simulink model "inv_pend_delay"  (Simulink 8.6)
settings: Solver=ode45  StartTime=0.0  StopTime=2  RelTol=1e-3
settings Model: Creator=mengg_000  LastModifiedBy=Martin
settings DebuggingCC: FcnCallInpInsideContextMsg=UseLocalSettings

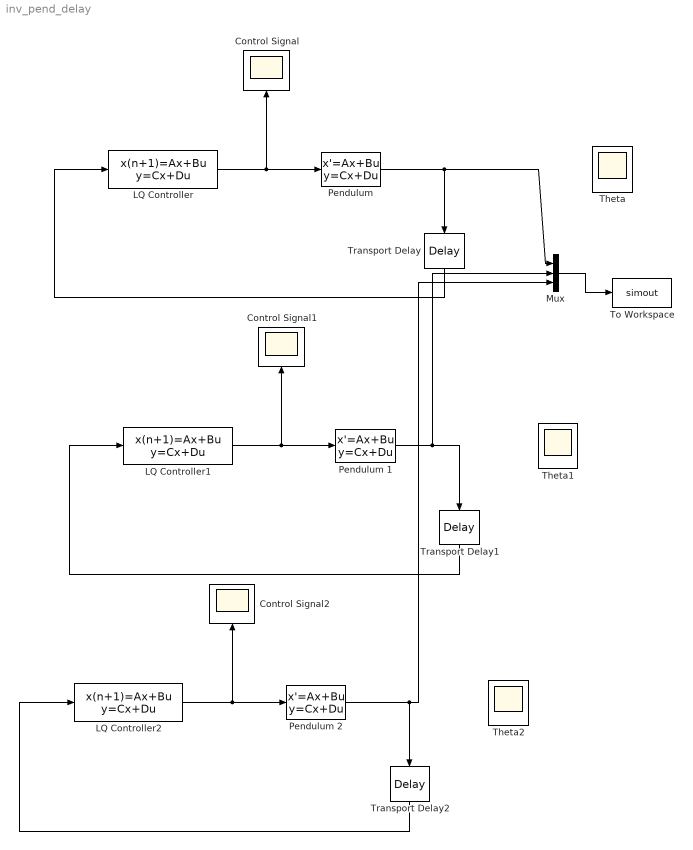
== system inv_pend_delay ==
  Control Signal : Scope
  Control Signal1 : Scope
  Control Signal2 : Scope
  LQ Controller : DiscreteStateSpace  A=|  B=|  C="[-12.1798  -13.3262         0]"  D=-8.1263  X0="[0;    0;   0]"  SampleTime=0.02
      A=|
      | [0.0389   -1.5001         0;
      |     0.0828    0.3594         0;
      |   -12.1798  -13.3262         0]
      B=|
      | [ -0.4344;
      |     0.1355;
      |    -8.1263]
  LQ Controller1 : DiscreteStateSpace  A=|  B=|  C="[-12.1798  -13.3262         0]"  D=-8.1263  X0="[0;    0;   0]"  SampleTime=0.02
      A=|
      | [0.0389   -1.5001         0;
      |     0.0828    0.3594         0;
      |   -12.1798  -13.3262         0]
      B=|
      | [ -0.4344;
      |     0.1355;
      |    -8.1263]
  LQ Controller2 : DiscreteStateSpace  A=|  B=|  C="[-12.1798  -13.3262         0]"  D=-8.1263  X0="[0;    0;   0]"  SampleTime=0.02
      A=|
      | [0.0389   -1.5001         0;
      |     0.0828    0.3594         0;
      |   -12.1798  -13.3262         0]
      B=|
      | [ -0.4344;
      |     0.1355;
      |    -8.1263]
  Mux : Mux  Inputs=3
  "Pendulum " : StateSpace  A=[0 3.0628;32 0]  B=[2; 0]  C=[0 1.5314]  D=0  X0=[0; 0.1]
  Pendulum 1 : StateSpace  A=[0 3.0628;32 0]  B=[2; 0]  C=[0 1.5314]  D=0  X0=[0; 0.1]
  Pendulum 2 : StateSpace  A=[0 3.0628;32 0]  B=[2; 0]  C=[0 1.5314]  D=0  X0=[0; 0.1]
  Theta : Scope
  Theta1 : Scope
  Theta2 : Scope
  To Workspace : ToWorkspace  VariableName=simout  SaveFormat=Timeseries  SampleTime=-1
  Transport Delay : TransportDelay  DelayTime=0.01
  Transport Delay1 : TransportDelay  DelayTime=0.04
  Transport Delay2 : TransportDelay  DelayTime=0.045
  wires:
  "Pendulum "/1 -> Mux/1, Transport Delay/1
  Transport Delay/1 -> LQ Controller/1
  LQ Controller/1 -> "Pendulum "/1, Control Signal/1
  Pendulum 1/1 -> Transport Delay1/1, Mux/2
  Transport Delay1/1 -> LQ Controller1/1
  LQ Controller1/1 -> Pendulum 1/1, Control Signal1/1
  Pendulum 2/1 -> Mux/3, Transport Delay2/1
  Transport Delay2/1 -> LQ Controller2/1
  LQ Controller2/1 -> Pendulum 2/1, Control Signal2/1
  Mux/1 -> To Workspace/1
